simulink model "gm_test_phase_voltages_without_delays"  (R2022a)
settings: Solver=FixedStepDiscrete  StartTime=0.0  StopTime=10.0  RelTol=1e-3
undefined symbols (not defined in the file or in its folder): f_c, u_dc
libraries: hdlmdlgenlib x22, simulink x2
(part 1 of 5)
settings Model: Creator=Andre Merx  LastModifiedBy=Andre Merx
settings SolverCC: AlgebraicLoopSolver=TrustRegion
settings DataIOCC: LimitDataPoints=on  SaveOutput=off  SaveTime=off
settings OptimizationCC: BlockReduction=off  ConditionallyExecuteInputs=off  DefaultParameterBehavior=Inlined  LifeSpan=inf
settings DebuggingCC: AlgebraicLoopMsg=error  InheritedTsInSrcMsg=none  SingleTaskRateTransMsg=error  UnconnectedInputMsg=warning  UnconnectedOutputMsg=warning  UnconnectedLineMsg=warning  AllowSymbolicDim=off  StrictBusMsg=ErrorOnBusTreatedAsVector  SFUnexpectedBacktrackingDiag=warning  SFNoUnconditionalDefaultTransitionDiag=warning  SFExecutionAtInitializationDiag=none  SFMachineParentedDataDiag=warning  ArithmeticOperatorsInVariantConditions=warning
settings HardwareCC: ProdBitPerPointer=32  ProdBitPerSizeT=32  ProdBitPerPtrDiffT=32  ProdLargestAtomicFloat=None  ProdIntDivRoundTo=Undefined  ProdEndianess=Unspecified  ProdWordSize=32  ProdHWDeviceType=ASIC/FPGA->ASIC/FPGA  ProdEqTarget=off
settings SFSimCC: SimUseLocalCustomCode=off  CustomCodeUndefinedFunction=UseInterfaceOnly
settings RTWCC: RTWUseLocalCustomCode=off
settings CodeAppCC: StateflowObjectComments=on
settings GRTTargetCC: TargetLangStandard=C89/C90 (ANSI)
settings ConfigComp: CovScope=ReferencedModels  CovMetricSettings=dw  CovSaveCumulativeToWorkspaceVar=on  CovSaveSingleToWorkspaceVar=on  CovExternalEMLEnable=off  CovSFcnEnable=off

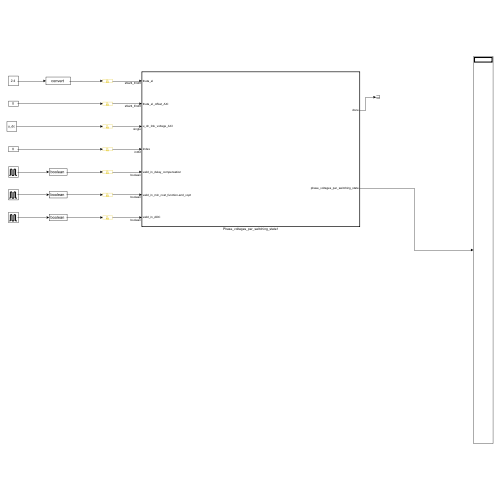
[thumbnail: Simulink's stored preview of the top-level diagram]
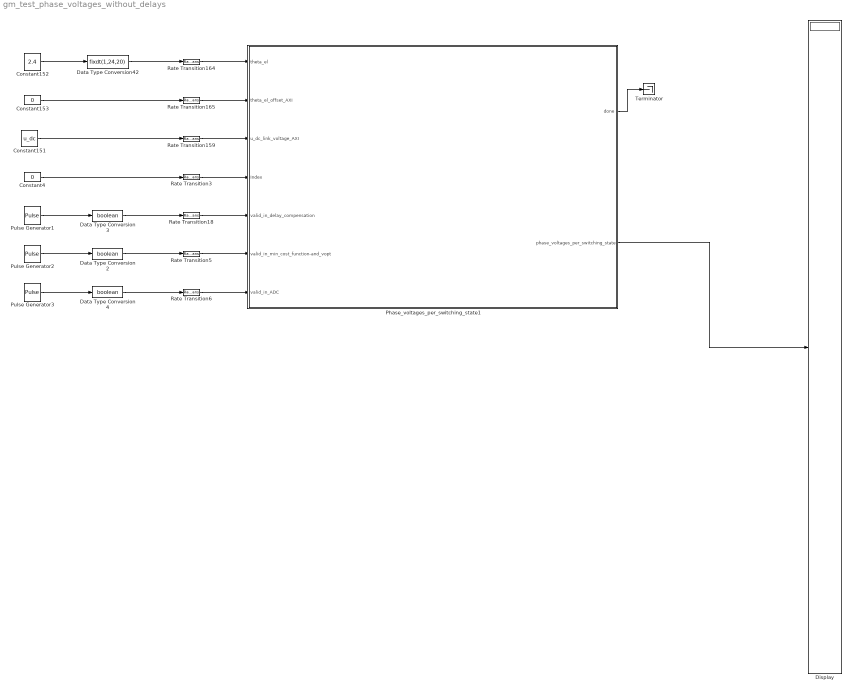
== system gm_test_phase_voltages_without_delays ==
  Constant151 : Constant  Value=u_dc  OutDataTypeStr=single  SampleTime=-1
  Constant152 : Constant  Value=2.4
  Constant153 : Constant  Value=0  OutDataTypeStr=fixdt(1,24,20)  SampleTime=-1
  Constant4 : Constant  Value=0  OutDataTypeStr=int32  SampleTime=-1
  Data Type Conversion2 : DataTypeConversion  OutDataTypeStr=boolean  SaturateOnIntegerOverflow=off  RndMeth=Floor
  Data Type Conversion3 : DataTypeConversion  OutDataTypeStr=boolean  SaturateOnIntegerOverflow=off  RndMeth=Floor
  Data Type Conversion4 : DataTypeConversion  OutDataTypeStr=boolean  SaturateOnIntegerOverflow=off  RndMeth=Floor
  Data Type Conversion42 : DataTypeConversion  OutDataTypeStr=fixdt(1,24,20)  SaturateOnIntegerOverflow=off  RndMeth=Floor
  Display : Display
  Phase_voltages_per_switching_state1 : Subsystem  TreatAsAtomicUnit=on
  Pulse Generator1 : DiscretePulseGenerator  PulseType=Time based  Period=1/f_c
  Pulse Generator2 : DiscretePulseGenerator  PulseType=Time based  Period=1/f_c
  Pulse Generator3 : DiscretePulseGenerator  PulseType=Time based  Period=1/f_c
  Rate Transition{3,5..6,18,159,164..165} (7 alike) : RateTransition  OutPortSampleTime=Rt
  Terminator : Terminator
  wires:
  Phase_voltages_per_switching_state1/2(phase_voltages_per_switching_state) -> Display/1
  Phase_voltages_per_switching_state1/1(done) -> Terminator/1
  Pulse Generator2/1 -> Data Type Conversion2/1
  Rate Transition5/1 -> Phase_voltages_per_switching_state1/6(valid_in_min_cost_function-and_vopt)
  Pulse Generator3/1 -> Data Type Conversion4/1
  Data Type Conversion2/1 -> Rate Transition5/1
  Constant4/1 -> Rate Transition3/1
  Data Type Conversion4/1 -> Rate Transition6/1
  Rate Transition3/1 -> Phase_voltages_per_switching_state1/4(Index)
  Pulse Generator1/1 -> Data Type Conversion3/1
  Rate Transition18/1 -> Phase_voltages_per_switching_state1/5(valid_in_delay_compensation)
  Rate Transition6/1 -> Phase_voltages_per_switching_state1/7(valid_in_ADC)
  Data Type Conversion3/1 -> Rate Transition18/1
  Data Type Conversion42/1 -> Rate Transition164/1
  Constant151/1 -> Rate Transition159/1
  Constant153/1 -> Rate Transition165/1
  Constant152/1 -> Data Type Conversion42/1
  Rate Transition159/1 -> Phase_voltages_per_switching_state1/3(u_dc_link_voltage_AXI)
  Rate Transition164/1 -> Phase_voltages_per_switching_state1/1(theta_el)
  Rate Transition165/1 -> Phase_voltages_per_switching_state1/2(theta_el_offset_AXI)

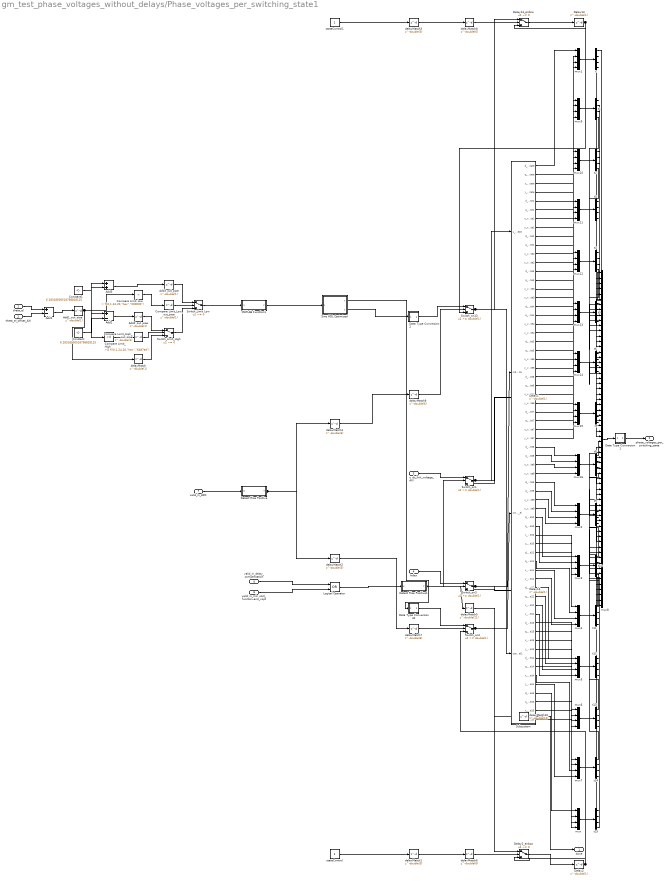
== system gm_test_phase_voltages_without_delays/Phase_voltages_per_switching_state1 ==
  theta_el : Inport  OutDataTypeStr=fixdt(1, 24, 20)  PortDimensions=1  SampleTime=1e-08
  theta_el_offset_AXI : Inport  Port=2  OutDataTypeStr=fixdt(1, 24, 20)  PortDimensions=1  SampleTime=1e-08
  u_dc_link_voltage_AXI : Inport  Port=3  OutDataTypeStr=single  PortDimensions=1  SampleTime=1e-08
  Index : Inport  Port=4  OutDataTypeStr=int32  PortDimensions=1  SampleTime=1e-08
  valid_in_delay_compensation : Inport  Port=5  OutDataTypeStr=boolean  PortDimensions=1  SampleTime=1e-08
  valid_in_min_cost_function-and_vopt : Inport  Port=6  OutDataTypeStr=boolean  PortDimensions=1  SampleTime=1e-08
  valid_in_ADC : Inport  Port=7  OutDataTypeStr=boolean  PortDimensions=1  SampleTime=1e-08
  Add1 : Sum  Inputs=+-  AccumDataTypeStr=fixdt(1, 24, 20)  OutDataTypeStr=fixdt(1, 24, 20)  SampleTime=1e-08
  Add1_out_pipe : Delay  DelayLength=double(1)  InitialCondition=0  SampleTime=1e-08
  Add2 : Sum  Inputs=+-  AccumDataTypeStr=fixdt(1, 24, 20)  OutDataTypeStr=fixdt(1, 24, 20)  SampleTime=1e-08
  Add2_out_pipe : Delay  DelayLength=double(1)  InitialCondition=0  SampleTime=1e-08
  Add3 : Sum  AccumDataTypeStr=fixdt(1, 24, 20)  OutDataTypeStr=fixdt(1, 24, 20)  SampleTime=1e-08
  Add3_out_pipe : Delay  DelayLength=double(1)  InitialCondition=0  SampleTime=1e-08
  Compare Limit_High : simulink/Logic and Bit Operations/Compare To Constant  relop=>=  const="fi(0,1,24,20,\"hex\",\"6487ed\")"  OutDataTypeStr=boolean
  Compare Limit_High_out_pipe : Delay  DelayLength=double(1)  InitialCondition=0  SampleTime=1e-08
  Compare Limit_Low : simulink/Logic and Bit Operations/Compare To Constant  relop=<  const="fi(0,1,24,20,\"hex\",\"000000\")"  OutDataTypeStr=boolean
  Compare Limit_Low_out_pipe : Delay  DelayLength=double(1)  InitialCondition=0  SampleTime=1e-08
  Constant : Constant  Value=6.28318500518798828125  OutDataTypeStr=fixdt(1, 24, 20)  SampleTime=1e-08
  Constant1 : Constant  Value=6.28318500518798828125  OutDataTypeStr=fixdt(1, 24, 20)  SampleTime=1e-08
  Data Type Conversion1 : Subsystem
      mask Display: disp('NFP\nconv');
  Data Type Conversion2 : Subsystem
      mask Display: disp('NFP\nconv');
  Data Type Conversion42 : Subsystem
      mask Display: disp('NFP\nconv');
  Delay{1..2,13..14} (4 alike) : Delay  DelayLength=double(1)  InitialCondition=0  SampleTime=1e-08
  Delay13_enbsw : Switch  Criteria=u2 ~= 0  Threshold=double(0)  OutDataTypeStr=single  SampleTime=1e-08  SaturateOnIntegerOverflow=off  InputSameDT=off
  Delay2_enbsw : Switch  Criteria=u2 ~= 0  Threshold=double(0)  OutDataTypeStr=single  SampleTime=1e-08  SaturateOnIntegerOverflow=off  InputSameDT=off
  Detect Rise Positive : Subsystem  mask(Detect Rise Positive){vinit=double(0), InputProcessing=Elements as channels (sample based), OutDataTypeStr=boolean}
      mask prompts: vinit "Simulink:masks:InitialCondition_MP"; InputProcessing "Simulink:masks:InputProcessing_MP"; OutDataTypeStr "Simulink:masks:OutputDataType_MP"
      mask help: Simulink:masks:DetectRisePositive_MD
      mask init:
      | InputProcessing = 'Elements as channels (sample based)';
      | OutDataTypeStr = 'boolean';
      | vinit = double(0);
      mask TypeOptions InputProcessing: Simulink:masks:ColumnsAsChannelsFrameBased | Simulink:masks:ElementsAsChannelsSampleBased
      mask TypeOptions OutDataTypeStr: Simulink:masks:uint8 | Simulink:masks:boolean
      mask Display: fprintf('U > 0\n&  NOT\nU/z > 0')
  Detect Rise Positive1 : Subsystem  mask(Detect Rise Positive){vinit=double(0), InputProcessing=Elements as channels (sample based), OutDataTypeStr=boolean}
      mask prompts: vinit "Simulink:masks:InitialCondition_MP"; InputProcessing "Simulink:masks:InputProcessing_MP"; OutDataTypeStr "Simulink:masks:OutputDataType_MP"
      mask help: Simulink:masks:DetectRisePositive_MD
      mask init:
      | InputProcessing = 'Elements as channels (sample based)';
      | OutDataTypeStr = 'boolean';
      | vinit = double(0);
      mask TypeOptions InputProcessing: Simulink:masks:ColumnsAsChannelsFrameBased | Simulink:masks:ElementsAsChannelsSampleBased
      mask TypeOptions OutDataTypeStr: Simulink:masks:uint8 | Simulink:masks:boolean
      mask Display: fprintf('U > 0\n&  NOT\nU/z > 0')
  Logical Operator : Logic  Operator=OR  AllPortsSameDT=off  OutDataTypeStr=boolean  SampleTime=1e-08
  MATLAB Function1 : Subsystem
  Sine HDL Optimized : Subsystem  mask(Sine and Cosine HDL optimized block){OutputFormula=sin(2*pi*u) and cos(2*pi*u), NumDataPoints=double(64), TableDataTypeStr=fixdt(1,24,20), SimulateLUTROMDelay=off}
      mask prompts: OutputFormula "Simulink:masks:OutputFormula_MP"; NumDataPoints "HDLShared:hdlshared:CosineHDL_Npts"; TableDataTypeStr "Simulink:blkprm_prompts:TABLE_UNIFIEDDATATYPE"; SimulateLUTROMDelay "HDLShared:hdlshared:CosineHDL_SimulateLUTDelay"
      mask help: Sine and Cosine HDL optimized block using quarter wave symmetry, and HDL friendly settings.
      mask Help: helpview([docroot '/hdlcoder/helptargets.map'],'SineAndCosineHDL_Optimized');
      mask TypeOptions OutputFormula: sin(2*pi*u) | cos(2*pi*u) | exp(j*2*pi*u) | sin(2*pi*u) and cos(2*pi*u)
      mask Display:
      | port_label('input',1,'u')
      | port_label('output',1,'sin(2*pi*u)')
      | port_label('output',2,'cos(2*pi*u)')
      | xpos = 0.35;
      | yoffset = 0.5;
      | if ( SimulateLUTROMDelay )
      |   text(xpos,yoffset,'HDL (Z^{-1})','texmode','on')
      | else
      |    text(xpos,yoffset,'HDL')
      | end
  Subsystem : Subsystem
  Switch_Limit_High : Switch  Criteria=u2 ~= 0  Threshold=double(0)  OutDataTypeStr=fixdt(1, 24, 20)  SampleTime=1e-08  SaturateOnIntegerOverflow=off  InputSameDT=off
  Switch_Limit_Low : Switch  Criteria=u2 ~= 0  Threshold=double(0)  OutDataTypeStr=fixdt(1, 24, 20)  SampleTime=1e-08  SaturateOnIntegerOverflow=off  InputSameDT=off
  Switch_on1 : Switch  Threshold=double(1)  OutDataTypeStr=single  RndMeth=Simplest  SampleTime=1e-08  SaturateOnIntegerOverflow=off  InputSameDT=off
  Switch_on13 : Switch  Threshold=double(1)  OutDataTypeStr=single  RndMeth=Simplest  SampleTime=1e-08  SaturateOnIntegerOverflow=off  InputSameDT=off
  Switch_on2 : Switch  Threshold=double(1)  OutDataTypeStr=single  RndMeth=Simplest  SampleTime=1e-08  SaturateOnIntegerOverflow=off  InputSameDT=off
  Switch_on3 : Switch  Threshold=double(1)  OutDataTypeStr=int32  RndMeth=Simplest  SampleTime=1e-08  SaturateOnIntegerOverflow=off  InputSameDT=off
  delayMatch : Delay  DelayLength=double(1)  InitialCondition=0  SampleTime=1e-08
  delayMatch{1..4} (4 alike) : Delay  DelayLength=double(3)  InitialCondition=0  SampleTime=1e-08
  delayMatch10 : Delay  DelayLength=double(12)  InitialCondition=0  SampleTime=1e-08
  delayMatch5 : Delay  DelayLength=double(21)  InitialCondition=0  SampleTime=1e-08
  delayMatch{6..9} (4 alike) : Delay  DelayLength=double(6)  InitialCondition=0  SampleTime=1e-08
  mux{,1..7,9..16} (16 alike) : Mux
  mux8 : Mux  Inputs=64
  stateControl : Constant  OutDataTypeStr=boolean  SampleTime=1e-08
  stateControl1 : Constant  OutDataTypeStr=boolean  SampleTime=1e-08
  t{,1..15} (16 alike) : Demux
  done : Outport  SampleTime=1e-08
  phase_voltages_per_switching_state : Outport  Port=2  SampleTime=1e-08
  wires:
  theta_el/1 -> Add1/1
  theta_el_offset_AXI/1 -> Add1/2
  u_dc_link_voltage_AXI/1 -> Switch_on1/1
  Index/1 -> Switch_on3/1
  valid_in_delay_compensation/1 -> Logical Operator/1
  valid_in_min_cost_function-and_vopt/1 -> Logical Operator/2
  valid_in_ADC/1 -> Detect Rise Positive/1(U)
  delayMatch/1 -> Switch_Limit_High/3
  Add2_out_pipe/1 -> Switch_Limit_High/1
  Add3_out_pipe/1 -> Switch_Limit_Low/1
  Compare Limit_High_out_pipe/1 -> Switch_Limit_High/2
  Compare Limit_Low_out_pipe/1 -> Switch_Limit_Low/2
  Constant/1 -> Add2/2
  Constant1/1 -> Add3/2
  delayMatch7/1 -> Switch_on2/2
  delayMatch10/1 -> done/1
  Logical Operator/1 -> Detect Rise Positive1/1(U)
  MATLAB Function1/1(y) -> Sine HDL Optimized/1(u)
  mux/1 -> t15/1
  mux1/1 -> t/1
  mux2/1 -> t9/1
  mux3/1 -> t10/1
  mux4/1 -> t11/1
  mux5/1 -> t12/1
  mux6/1 -> t13/1
  mux7/1 -> t14/1
  mux8/1 -> Data Type Conversion1/1(In1)
  mux9/1 -> t1/1
  mux10/1 -> t2/1
  mux11/1 -> t3/1
  mux12/1 -> t4/1
  mux13/1 -> t5/1
  mux14/1 -> t6/1
  mux15/1 -> t7/1
  mux16/1 -> t8/1
  Sine HDL Optimized/1(x) -> Data Type Conversion42/1(In1)
  Sine HDL Optimized/2(y) -> Data Type Conversion2/1(In1)
  Subsystem/1(d_voltage_per_switching_state) -> mux1/1
  Subsystem/2(q_voltage_per_switching_state) -> mux1/2
  Subsystem/3(x_voltage_per_switching_state) -> mux1/3
  Subsystem/4(y_voltage_per_switching_state) -> mux1/4
  Subsystem/5(d_voltage_per_switching_state1) -> mux9/1
  Subsystem/6(q_voltage_per_switching_state1) -> mux9/2
  Subsystem/7(x_voltage_per_switching_state1) -> mux9/3
  Subsystem/8(y_voltage_per_switching_state1) -> mux9/4
  Subsystem/9(d_voltage_per_switching_state2) -> mux10/1
  Subsystem/10(q_voltage_per_switching_state2) -> mux10/2
  Subsystem/11(x_voltage_per_switching_state2) -> mux10/3
  Subsystem/12(y_voltage_per_switching_state2) -> mux10/4
  Subsystem/13(d_voltage_per_switching_state3) -> mux11/1
  Subsystem/14(q_voltage_per_switching_state3) -> mux11/2
  Subsystem/15(x_voltage_per_switching_state3) -> mux11/3
  Subsystem/16(y_voltage_per_switching_state3) -> mux11/4
  Subsystem/17(d_voltage_per_switching_state4) -> mux12/1
  Subsystem/18(q_voltage_per_switching_state4) -> mux12/2
  Subsystem/19(x_voltage_per_switching_state4) -> mux12/3
  Subsystem/20(y_voltage_per_switching_state4) -> mux12/4
  Subsystem/21(d_voltage_per_switching_state5) -> mux13/1
  Subsystem/22(q_voltage_per_switching_state5) -> mux13/2
  Subsystem/23(x_voltage_per_switching_state5) -> mux13/3
  Subsystem/24(y_voltage_per_switching_state5) -> mux13/4
  Subsystem/25(d_voltage_per_switching_state6) -> mux14/1
  Subsystem/26(q_voltage_per_switching_state6) -> mux14/2
  Subsystem/27(x_voltage_per_switching_state6) -> mux14/3
  Subsystem/28(y_voltage_per_switching_state6) -> mux14/4
  Subsystem/29(d_voltage_per_switching_state7) -> mux15/1
  Subsystem/30(q_voltage_per_switching_state7) -> mux15/2
  Subsystem/31(x_voltage_per_switching_state7) -> mux15/3
  Subsystem/32(y_voltage_per_switching_state7) -> mux15/4
  Subsystem/33(d_voltage_per_switching_state8) -> mux16/1
  Subsystem/34(q_voltage_per_switching_state8) -> mux16/2
  Subsystem/35(x_voltage_per_switching_state8) -> mux16/3
  Subsystem/36(y_voltage_per_switching_state8) -> mux16/4
  Subsystem/37(d_voltage_per_switching_state9) -> mux2/1
  Subsystem/38(q_voltage_per_switching_state9) -> mux2/2
  Subsystem/39(x_voltage_per_switching_state9) -> mux2/3
  Subsystem/40(y_voltage_per_switching_state9) -> mux2/4
  Subsystem/41(d_voltage_per_switching_state10) -> mux3/1
  Subsystem/42(q_voltage_per_switching_state10) -> mux3/2
  Subsystem/43(x_voltage_per_switching_state10) -> mux3/3
  Subsystem/44(y_voltage_per_switching_state10) -> mux3/4
  Subsystem/45(d_voltage_per_switching_state11) -> mux4/1
  Subsystem/46(q_voltage_per_switching_state11) -> mux4/2
  Subsystem/47(x_voltage_per_switching_state11) -> mux4/3
  Subsystem/48(y_voltage_per_switching_state11) -> mux4/4
  Subsystem/49(d_voltage_per_switching_state12) -> mux5/1
  Subsystem/50(q_voltage_per_switching_state12) -> mux5/2
  Subsystem/51(x_voltage_per_switching_state12) -> mux5/3
  Subsystem/52(y_voltage_per_switching_state12) -> mux5/4
  Subsystem/53(d_voltage_per_switching_state13) -> mux6/1
  Subsystem/54(q_voltage_per_switching_state13) -> mux6/2
  Subsystem/55(x_voltage_per_switching_state13) -> mux6/3
  Subsystem/56(y_voltage_per_switching_state13) -> mux6/4
  Subsystem/57(d_voltage_per_switching_state14) -> mux7/1
  Subsystem/58(q_voltage_per_switching_state14) -> mux7/2
  Subsystem/59(x_voltage_per_switching_state14) -> mux7/3
  Subsystem/60(y_voltage_per_switching_state14) -> mux7/4
  Subsystem/61(d_voltage_per_switching_state15) -> mux/1
  Subsystem/62(q_voltage_per_switching_state15) -> mux/2
  Subsystem/63(x_voltage_per_switching_state15) -> mux/3
  Subsystem/64(y_voltage_per_switching_state15) -> mux/4
  Switch_Limit_High/1 -> Switch_Limit_Low/3
  Switch_Limit_Low/1 -> MATLAB Function1/1(u)
  Switch_on1/1 -> Subsystem/1(u_dc_link_voltage15), Delay1/1
  Switch_on3/1 -> Subsystem/2(Index 15), Delay14/1
  Add1/1 -> Add1_out_pipe/1
  Add2/1 -> Add2_out_pipe/1
  Add3/1 -> Add3_out_pipe/1
  Compare Limit_High/1 -> Compare Limit_High_out_pipe/1
  Compare Limit_Low/1 -> Compare Limit_Low_out_pipe/1
  t/1 -> mux8/1
  t/2 -> mux8/2
  t/3 -> mux8/3
  t/4 -> mux8/4
  t1/1 -> mux8/5
  t1/2 -> mux8/6
  t1/3 -> mux8/7
  t1/4 -> mux8/8
  t2/1 -> mux8/9
  t2/2 -> mux8/10
  t2/3 -> mux8/11
  t2/4 -> mux8/12
  t3/1 -> mux8/13
  t3/2 -> mux8/14
  t3/3 -> mux8/15
  t3/4 -> mux8/16
  t4/1 -> mux8/17
  t4/2 -> mux8/18
  t4/3 -> mux8/19
  t4/4 -> mux8/20
  t5/1 -> mux8/21
  t5/2 -> mux8/22
  t5/3 -> mux8/23
  t5/4 -> mux8/24
  t6/1 -> mux8/25
  t6/2 -> mux8/26
  t6/3 -> mux8/27
  t6/4 -> mux8/28
  t7/1 -> mux8/29
  t7/2 -> mux8/30
  t7/3 -> mux8/31
  t7/4 -> mux8/32
  t8/1 -> mux8/33
  t8/2 -> mux8/34
  t8/3 -> mux8/35
  t8/4 -> mux8/36
  t9/1 -> mux8/37
  t9/2 -> mux8/38
  t9/3 -> mux8/39
  t9/4 -> mux8/40
  t10/1 -> mux8/41
  t10/2 -> mux8/42
  t10/3 -> mux8/43
  t10/4 -> mux8/44
  t11/1 -> mux8/45
  t11/2 -> mux8/46
  t11/3 -> mux8/47
  t11/4 -> mux8/48
  t12/1 -> mux8/49
  t12/2 -> mux8/50
  t12/3 -> mux8/51
  t12/4 -> mux8/52
  t13/1 -> mux8/53
  t13/2 -> mux8/54
  t13/3 -> mux8/55
  t13/4 -> mux8/56
  t14/1 -> mux8/57
  t14/2 -> mux8/58
  t14/3 -> mux8/59
  t14/4 -> mux8/60
  t15/1 -> mux8/61
  t15/2 -> mux8/62
  t15/3 -> mux8/63
  t15/4 -> mux8/64
  delayMatch6/1 -> Delay2_enbsw/2
  delayMatch8/1 -> Delay13_enbsw/2
  Add1_out_pipe/1 -> delayMatch/1, Compare Limit_Low/1, Compare Limit_High/1, Add3/1, Add2/1
  stateControl/1 -> delayMatch1/1
  delayMatch9/1 -> Switch_on13/2
  stateControl1/1 -> delayMatch3/1
  Detect Rise Positive/1(Y) -> delayMatch4/1, delayMatch2/1
  Detect Rise Positive1/1(Y) -> delayMatch5/1, Switch_on1/2, Switch_on3/2
  Data Type Conversion1/1(Out1) -> phase_voltages_per_switching_state/1
  Data Type Conversion2/1(Out1) -> Switch_on13/1
  Data Type Conversion42/1(Out1) -> Switch_on2/1
  delayMatch1/1 -> delayMatch6/1
  delayMatch2/1 -> delayMatch7/1
  delayMatch3/1 -> delayMatch8/1
  delayMatch4/1 -> delayMatch9/1
  delayMatch5/1 -> delayMatch10/1
  Switch_on2/1 -> Subsystem/3(sin_theta_el), Delay2_enbsw/1
  Switch_on13/1 -> Subsystem/4(cos_theta_el1), Delay13_enbsw/1
  Delay1/1 -> Switch_on1/3
  Delay14/1 -> Switch_on3/3
  Delay2_enbsw/1 -> Delay2/1
  Delay2/1 -> Switch_on2/3, Delay2_enbsw/3
  Delay13_enbsw/1 -> Delay13/1
  Delay13/1 -> Switch_on13/3, Delay13_enbsw/3

== system gm_test_phase_voltages_without_delays/Phase_voltages_per_switching_state1/Data Type Conversion1 ==
  In1 : Inport
  Data Type Conversion1 : DataTypeConversion  OutDataTypeStr=fixdt(1, 24, 11)  SampleTime=1e-08  SaturateOnIntegerOverflow=off  RndMeth=Floor
  Data Type Conversion1_pd1 : Delay  DelayLength=6
  Out1 : Outport
  wires:
  In1/1 -> Data Type Conversion1/1
  Data Type Conversion1/1 -> Data Type Conversion1_pd1/1
  Data Type Conversion1_pd1/1 -> Out1/1

== system gm_test_phase_voltages_without_delays/Phase_voltages_per_switching_state1/Data Type Conversion2 ==
  In1 : Inport
  Data Type Conversion2 : DataTypeConversion  OutDataTypeStr=single  SampleTime=1e-08  SaturateOnIntegerOverflow=off  RndMeth=Floor
  Data Type Conversion2_pd1 : Delay  DelayLength=6
  Out1 : Outport
  wires:
  In1/1 -> Data Type Conversion2/1
  Data Type Conversion2/1 -> Data Type Conversion2_pd1/1
  Data Type Conversion2_pd1/1 -> Out1/1

== system gm_test_phase_voltages_without_delays/Phase_voltages_per_switching_state1/Data Type Conversion42 ==
  In1 : Inport
  Data Type Conversion42 : DataTypeConversion  OutDataTypeStr=single  SampleTime=1e-08  SaturateOnIntegerOverflow=off  RndMeth=Floor
  Data Type Conversion42_pd1 : Delay  DelayLength=6
  Out1 : Outport
  wires:
  In1/1 -> Data Type Conversion42/1
  Data Type Conversion42/1 -> Data Type Conversion42_pd1/1
  Data Type Conversion42_pd1/1 -> Out1/1

== system gm_test_phase_voltages_without_delays/Phase_voltages_per_switching_state1/Detect Rise Positive ==
  note: Edge
  note: U(k)
  U : Inport  OutDataTypeStr=boolean  SampleTime=1e-08
  Delay Input1 : UnitDelay  Description=Store in Global RAM  DisableCoverage=on  InitialCondition=vinit  SampleTime=-1  HasFrameUpgradeWarning=on
  FixPt Relational Operator : RelationalOperator  Operator=>  OutDataTypeStr=boolean  ZeroCross=off  InputSameDT=off
  Positive : Subsystem  mask(Compare To Zero){relop=>, OutDataTypeStr=boolean, ZeroCross=off}
      mask prompts: relop "Simulink:masks:Operator_MP"; OutDataTypeStr "Simulink:masks:OutputDataType_MP"; ZeroCross "Simulink:masks:EnableZerocrossingDetection_MP"
      mask help: Simulink:masks:CompareToZero_MD
      mask init:
      | OutDataTypeStr = 'boolean';
      | ZeroCross = 'off';
      | blkName = 'test_phase_voltages_without_delays/Phase_voltages_per_switching_state1/Detect Rise\nPositive/Positive';
      | relop = '>';
      | setValue = 'boolean';
      mask TypeOptions relop: == | ~= | < | <= | >= | >
      mask TypeOptions OutDataTypeStr: Simulink:masks:uint8 | Simulink:masks:boolean
      mask Callback ZeroCross: sl('zeroCrossEnable', gcbh);
      mask Display: disp([relop,' 0'])
  Y : Outport  SampleTime=1e-08
  wires:
  Delay Input1/1 -> FixPt Relational Operator/2
  FixPt Relational Operator/1 -> Y/1
  Positive/1(y) -> FixPt Relational Operator/1, Delay Input1/1
  U/1 -> Positive/1(u)

== system gm_test_phase_voltages_without_delays/Phase_voltages_per_switching_state1/Detect Rise Positive1 ==
  note: Edge
  note: U(k)
  U : Inport  OutDataTypeStr=boolean  SampleTime=1e-08
  Delay Input1 : UnitDelay  Description=Store in Global RAM  DisableCoverage=on  InitialCondition=vinit  SampleTime=-1  HasFrameUpgradeWarning=on
  FixPt Relational Operator : RelationalOperator  Operator=>  OutDataTypeStr=boolean  ZeroCross=off  InputSameDT=off
  Positive : Subsystem  mask(Compare To Zero){relop=>, OutDataTypeStr=boolean, ZeroCross=off}
      mask prompts: relop "Simulink:masks:Operator_MP"; OutDataTypeStr "Simulink:masks:OutputDataType_MP"; ZeroCross "Simulink:masks:EnableZerocrossingDetection_MP"
      mask help: Simulink:masks:CompareToZero_MD
      mask init:
      | OutDataTypeStr = 'boolean';
      | ZeroCross = 'off';
      | blkName = 'test_phase_voltages_without_delays/Phase_voltages_per_switching_state1/Detect Rise\nPositive1/Positive';
      | relop = '>';
      | setValue = 'boolean';
      mask TypeOptions relop: == | ~= | < | <= | >= | >
      mask TypeOptions OutDataTypeStr: Simulink:masks:uint8 | Simulink:masks:boolean
      mask Callback ZeroCross: sl('zeroCrossEnable', gcbh);
      mask Display: disp([relop,' 0'])
  Y : Outport  SampleTime=1e-08
  wires:
  Delay Input1/1 -> FixPt Relational Operator/2
  FixPt Relational Operator/1 -> Y/1
  Positive/1(y) -> FixPt Relational Operator/1, Delay Input1/1
  U/1 -> Positive/1(u)

== system gm_test_phase_voltages_without_delays/Phase_voltages_per_switching_state1/MATLAB Function1 ==
  u : Inport  OutDataTypeStr=fixdt(1, 24, 20)  PortDimensions=1  SampleTime=1e-08
  MATLAB Function1 : MATLAB Function  TreatAsAtomicUnit=on
  y : Outport  SampleTime=1e-08  VectorParamsAs1DForOutWhenUnconnected=off
  wires:
  MATLAB Function1/1(y) -> y/1
  u/1 -> MATLAB Function1/1(u)

== system gm_test_phase_voltages_without_delays/Phase_voltages_per_switching_state1/Sine HDL Optimized ==
  note: (C) 2016 Mathworks, Inc
  note: (C) 2016 Mathworks, Inc
  u : Inport  OutDataTypeStr=fixdt(1,48,45,'DataTypeOverride', 'Off')  SampleTime=1e-08
  1st or 4th Quad : Logic  Operator=OR  AllPortsSameDT=off  OutDataTypeStr=boolean  SampleTime=1e-08
  Amp25 : Sum  Inputs=+-  AccumDataTypeStr=fixdt(1, 26, 25)  OutDataTypeStr=fixdt(1, 26, 25)  SampleTime=1e-08
  Amp50 : Sum  Inputs=+-  AccumDataTypeStr=fixdt(1, 26, 25)  OutDataTypeStr=fixdt(1, 26, 25)  SampleTime=1e-08
  Amp75 : Sum  Inputs=+-  AccumDataTypeStr=fixdt(1, 26, 25)  OutDataTypeStr=fixdt(1, 26, 25)  SampleTime=1e-08
  CastU16En1 : DataTypeConversion  OutDataTypeStr=uint8  ConvertRealWorld=Stored Integer (SI)  SampleTime=1e-08  SaturateOnIntegerOverflow=off  RndMeth=Floor
  CastU16En2 : DataTypeConversion  OutDataTypeStr=uint8  ConvertRealWorld=Stored Integer (SI)  SampleTime=1e-08  RndMeth=Floor
  CastU16En21 : DataTypeConversion  OutDataTypeStr=uint8  ConvertRealWorld=Stored Integer (SI)  SampleTime=1e-08  SaturateOnIntegerOverflow=off  RndMeth=Floor
  CastU16En3 : DataTypeConversion  OutDataTypeStr=fixdt(0, 9, 0)  SampleTime=1e-08  SaturateOnIntegerOverflow=off  RndMeth=Floor
  CastU16En31 : DataTypeConversion  OutDataTypeStr=uint8  ConvertRealWorld=Stored Integer (SI)  SampleTime=1e-08  RndMeth=Floor
  CastU16En4 : DataTypeConversion  OutDataTypeStr=fixdt(0, 9, 0)  SampleTime=1e-08  SaturateOnIntegerOverflow=off  RndMeth=Floor
  Cosine : hdlmdlgenlib/Buffer
      settings: SourceProductBaseCode=SL
  Cosine1 : hdlmdlgenlib/Buffer
      settings: SourceProductBaseCode=SL
  GTEp75 : RelationalOperator  OutDataTypeStr=boolean  SampleTime=1e-08  InputSameDT=off
  LTEp{25,50,251,501} (4 alike) : RelationalOperator  Operator=<=  OutDataTypeStr=boolean  SampleTime=1e-08  InputSameDT=off
  Look-Up Table : Lookup_n-D  NumberOfTableDimensions=1  BreakpointsForDimension1="fi(\"numerictype\",numerictype(0,8,0),\"fimath\",fimath(\"RoundingMethod\", \"Floor\",\"OverflowAction\", \"Wrap\",\"ProductMode\",\"FullPrecision\",\"SumMode\",\"FullPrecision\"),\"Value\",\"[0 1 2 3 4 5 6 7 8 9 10 11 12 13 14 15 16 17 18 19 20 21 22 23 24 25 26 27 28 29 30 31 32 33 34 35 36 37 38 39 40 41 42 43 44 45 46 47 48 49 50 51 52 53 54 55 56 57 58 59 60 61 62 63]\")"  Table="reshape(fi(\"numerictype\",numerictype(1,25,20),\"fimath\",fimath(\"RoundingMethod\", \"Floor\",\"OverflowAction\", \"Wrap\",\"ProductMode\",\"FullPrecision\",\"SumMode\",\"FullPrecision\"),\"Value\",\"[0;0.02454090118408203125;0.04906749725341796875;0.0735645294189453125;0.0980167388916015625;0.12241077423095703125;0.1467304229736328125;0.17096233367919921875;0.19509029388427734375;0.2191009521484375;0.24298000335693359375;0.26671314239501953125;0.2902851104736328125;0.31368160247802734375;0.33689022064208984375;0.35989475250244140625;0.38268375396728515625;0.4052410125732421875;0.427555084228515625;0.449611663818359375;0.47139644622802734375;0.49289798736572265625;0.514102935791015625;0.5349979400634765625;0.5555706024169921875;0.57580852508544921875;0.595699310302734375;0.61523151397705078125;0.6343936920166015625;0.65317249298095703125;0.67155933380126953125;0.689540863037109375;0.70710659027099609375;0.724246978759765625;0.7409515380859375;0.75720882415771484375;0.77301025390625;0.78834629058837890625;0.8032073974609375;0.817584991455078125;0.83146953582763671875;0.84485340118408203125;0.8577289581298828125;0.870086669921875;0.88192081451416015625;0.8932247161865234375;0.90398883819580078125;0.9142093658447265625;0.9238796234130859375;0.9329929351806640625;0.94154453277587890625;0.949527740478515625;0.95694065093994140625;0.963775634765625;0.97003078460693359375;0.9757022857666015625;0.980785369873046875;0.9852771759033203125;0.98917675018310546875;0.9924793243408203125;0.99518489837646484375;0.99729061126708984375;0.99879550933837890625;0.999698638916015625]\"), [1  64])"  InterpMethod=Flat  ExtrapMethod=Clip  DiagnosticForOutOfRangeInput=Error  SampleTime=1e-08  OutDataTypeStr=fixdt(1, 25, 20)
  Look-Up Table1 : Lookup_n-D  NumberOfTableDimensions=1  BreakpointsForDimension1="fi(\"numerictype\",numerictype(0,8,0),\"fimath\",fimath(\"RoundingMethod\", \"Floor\",\"OverflowAction\", \"Wrap\",\"ProductMode\",\"FullPrecision\",\"SumMode\",\"FullPrecision\"),\"Value\",\"[0 1 2 3 4 5 6 7 8 9 10 11 12 13 14 15 16 17 18 19 20 21 22 23 24 25 26 27 28 29 30 31 32 33 34 35 36 37 38 39 40 41 42 43 44 45 46 47 48 49 50 51 52 53 54 55 56 57 58 59 60 61 62 63]\")"  Table="reshape(fi(\"numerictype\",numerictype(1,25,20),\"fimath\",fimath(\"RoundingMethod\", \"Floor\",\"OverflowAction\", \"Wrap\",\"ProductMode\",\"FullPrecision\",\"SumMode\",\"FullPrecision\"),\"Value\",\"[0;0.02454090118408203125;0.04906749725341796875;0.0735645294189453125;0.0980167388916015625;0.12241077423095703125;0.1467304229736328125;0.17096233367919921875;0.19509029388427734375;0.2191009521484375;0.24298000335693359375;0.26671314239501953125;0.2902851104736328125;0.31368160247802734375;0.33689022064208984375;0.35989475250244140625;0.38268375396728515625;0.4052410125732421875;0.427555084228515625;0.449611663818359375;0.47139644622802734375;0.49289798736572265625;0.514102935791015625;0.5349979400634765625;0.5555706024169921875;0.57580852508544921875;0.595699310302734375;0.61523151397705078125;0.6343936920166015625;0.65317249298095703125;0.67155933380126953125;0.689540863037109375;0.70710659027099609375;0.724246978759765625;0.7409515380859375;0.75720882415771484375;0.77301025390625;0.78834629058837890625;0.8032073974609375;0.817584991455078125;0.83146953582763671875;0.84485340118408203125;0.8577289581298828125;0.870086669921875;0.88192081451416015625;0.8932247161865234375;0.90398883819580078125;0.9142093658447265625;0.9238796234130859375;0.9329929351806640625;0.94154453277587890625;0.949527740478515625;0.95694065093994140625;0.963775634765625;0.97003078460693359375;0.9757022857666015625;0.980785369873046875;0.9852771759033203125;0.98917675018310546875;0.9924793243408203125;0.99518489837646484375;0.99729061126708984375;0.99879550933837890625;0.999698638916015625]\"), [1  64])"  InterpMethod=Flat  ExtrapMethod=Clip  DiagnosticForOutOfRangeInput=Error  SampleTime=1e-08  OutDataTypeStr=fixdt(1, 25, 20)
  Negate : UnaryMinus  SampleTime=1e-08
  Negate1 : UnaryMinus  SampleTime=1e-08
  PipelineRegister : Delay  DelayLength=double(1)  InitialCondition=0  SampleTime=1e-08
  PipelineRegister1 : Delay  DelayLength=double(1)  InitialCondition=0  SampleTime=1e-08
  Point25 : Constant  Value=0.25  OutDataTypeStr=fixdt(0, 25, 25)  SampleTime=1e-08
  Point251 : Constant  Value=0.25  OutDataTypeStr=fixdt(0, 25, 25)  SampleTime=1e-08
  Point50 : Constant  Value=0.5  OutDataTypeStr=fixdt(0, 25, 25)  SampleTime=1e-08
  Point501 : Constant  Value=0.5  OutDataTypeStr=fixdt(0, 25, 25)  SampleTime=1e-08
  Point75 : Constant  Value=0.75  OutDataTypeStr=fixdt(0, 25, 25)  SampleTime=1e-08
  Positive : DataTypeConversion  OutDataTypeStr=fixdt(1, 25, 20)  SampleTime=1e-08  SaturateOnIntegerOverflow=off  RndMeth=Floor
  Positive1 : DataTypeConversion  OutDataTypeStr=fixdt(1, 25, 20)  SampleTime=1e-08  SaturateOnIntegerOverflow=off  RndMeth=Floor
  QuadHandle1 : Switch  Criteria=u2 ~= 0  Threshold=double(0)  OutDataTypeStr=fixdt(1, 26, 25)  SampleTime=1e-08  SaturateOnIntegerOverflow=off  InputSameDT=off
  QuadHandle1a : Switch  Criteria=u2 ~= 0  Threshold=double(0)  OutDataTypeStr=fixdt(1, 26, 25)  SampleTime=1e-08  SaturateOnIntegerOverflow=off  InputSameDT=off
  QuadHandle1b : Switch  Criteria=u2 ~= 0  Threshold=double(0)  OutDataTypeStr=fixdt(1, 26, 25)  SampleTime=1e-08  SaturateOnIntegerOverflow=off  InputSameDT=off
  QuadHandle2 : Switch  Criteria=u2 ~= 0  Threshold=double(0)  OutDataTypeStr=fixdt(0, 8, 8)  SampleTime=1e-08  InputSameDT=off
  QuadHandle21 : Switch  Criteria=u2 ~= 0  Threshold=double(0)  OutDataTypeStr=fixdt(0, 8, 8)  SampleTime=1e-08  SaturateOnIntegerOverflow=off  InputSameDT=off
  RAMDelayBalance : hdlmdlgenlib/Buffer
      settings: SourceProductBaseCode=SL
  RAMDelayBalance1 : hdlmdlgenlib/Buffer
      settings: SourceProductBaseCode=SL
  Saturation : Saturate  UpperLimit="fi(0,0,8,0,\"hex\",\"3f\")"  LowerLimit="fi(0,0,8,0,\"hex\",\"00\")"  SampleTime=1e-08  OutDataTypeStr=uint8
  Saturation1 : Saturate  UpperLimit="fi(0,0,8,0,\"hex\",\"3f\")"  LowerLimit="fi(0,0,8,0,\"hex\",\"00\")"  SampleTime=1e-08  OutDataTypeStr=uint8
  SignCorrected : Switch  Criteria=u2 ~= 0  Threshold=double(0)  OutDataTypeStr=fixdt(1, 25, 20)  SampleTime=1e-08  SaturateOnIntegerOverflow=off  InputSameDT=off
  SignCorrected1 : Switch  Criteria=u2 ~= 0  Threshold=double(0)  OutDataTypeStr=fixdt(1, 25, 20)  SampleTime=1e-08  SaturateOnIntegerOverflow=off  InputSameDT=off
  Sine : hdlmdlgenlib/Buffer
      settings: SourceProductBaseCode=SL
  Sine1 : hdlmdlgenlib/Buffer
      settings: SourceProductBaseCode=SL
  Switch : Switch  Criteria=u2 ~= 0  Threshold=double(0)  OutDataTypeStr=uint8  SampleTime=1e-08  SaturateOnIntegerOverflow=off  InputSameDT=off
  Switch1 : Switch  Criteria=u2 ~= 0  Threshold=double(0)  OutDataTypeStr=uint8  SampleTime=1e-08  SaturateOnIntegerOverflow=off  InputSameDT=off
  delayMatch : Delay  DelayLength=double(1)  InitialCondition=0  SampleTime=1e-08
  delayMatch1 : Delay  DelayLength=double(1)  InitialCondition=0  SampleTime=1e-08
  dtc : DataTypeConversion  OutDataTypeStr=uint8  SampleTime=1e-08  SaturateOnIntegerOverflow=off  RndMeth=Floor
  insig : DataTypeConversion  OutDataTypeStr=fixdt(0, 8, 8)  SampleTime=1e-08  SaturateOnIntegerOverflow=off  RndMeth=Floor
  insig1 : DataTypeConversion  OutDataTypeStr=fixdt(0, 8, 8)  SampleTime=1e-08  SaturateOnIntegerOverflow=off  RndMeth=Floor
  p25mA : Sum  Inputs=+-  AccumDataTypeStr=fixdt(1, 26, 25)  OutDataTypeStr=fixdt(1, 26, 25)  SampleTime=1e-08
  p50mA : Sum  Inputs=+-  AccumDataTypeStr=fixdt(1, 27, 25)  OutDataTypeStr=fixdt(1, 27, 25)  SampleTime=1e-08
  p75mA : Sum  Inputs=+-  AccumDataTypeStr=fixdt(1, 26, 25)  OutDataTypeStr=fixdt(1, 26, 25)  SampleTime=1e-08
  pow2switch : Constant  OutDataTypeStr=boolean  SampleTime=1e-08
  pow2switch1 : Constant  OutDataTypeStr=boolean  SampleTime=1e-08
  x : Outport  SampleTime=1e-08
  y : Outport  Port=2  SampleTime=1e-08
  wires:
  Sine1/1 -> x/1
  Cosine1/1 -> y/1
  Cosine/1 -> Cosine1/1
  Sine/1 -> Sine1/1
  dtc/1 -> RAMDelayBalance/1
  Amp25/1 -> QuadHandle1a/3
  Amp75/1 -> QuadHandle1b/1
  CastU16En1/1 -> CastU16En3/1
  CastU16En2/1 -> Switch/3, Saturation/1
  CastU16En3/1 -> CastU16En2/1
  GTEp75/1 -> QuadHandle1b/2, 1st or 4th Quad/2
  LTEp25/1 -> QuadHandle1a/2, 1st or 4th Quad/1
  LTEp50/1 -> QuadHandle2/2
  PipelineRegister/1 -> Positive/1, Negate/1
  Negate/1 -> SignCorrected/3
  Point25/1 -> p25mA/1, LTEp25/2, Amp25/2
  Point50/1 -> LTEp50/2
  Point75/1 -> p75mA/1, GTEp75/2, Amp75/2
  Positive/1 -> SignCorrected/1
  QuadHandle1a/1 -> QuadHandle2/1
  QuadHandle1b/1 -> QuadHandle2/3
  QuadHandle2/1 -> CastU16En1/1
  delayMatch1/1 -> SignCorrected/2
  Saturation/1 -> Switch/1
  SignCorrected/1 -> Cosine/1
  Switch/1 -> Look-Up Table/1
  insig/1 -> p75mA/2, p25mA/2, LTEp50/1, LTEp25/1, GTEp75/1, Amp75/1, Amp25/1
  p25mA/1 -> QuadHandle1a/1
  p75mA/1 -> QuadHandle1b/3
  pow2switch/1 -> Switch/2
  Amp50/1 -> QuadHandle1/3
  CastU16En21/1 -> CastU16En4/1
  CastU16En31/1 -> Switch1/3, Saturation1/1
  CastU16En4/1 -> CastU16En31/1
  LTEp251/1 -> QuadHandle21/2
  LTEp501/1 -> QuadHandle1/2, RAMDelayBalance1/1
  PipelineRegister1/1 -> Positive1/1, Negate1/1
  Negate1/1 -> SignCorrected1/3
  Point251/1 -> LTEp251/2
  Point501/1 -> p50mA/1, LTEp501/2, Amp50/2
  Positive1/1 -> SignCorrected1/1
  QuadHandle1/1 -> p50mA/2, QuadHandle21/1, LTEp251/1
  QuadHandle21/1 -> CastU16En21/1
  delayMatch/1 -> SignCorrected1/2
  Saturation1/1 -> Switch1/1
  SignCorrected1/1 -> Sine/1
  Switch1/1 -> Look-Up Table1/1
  insig1/1 -> QuadHandle1/1, LTEp501/1, Amp50/1
  p50mA/1 -> QuadHandle21/3
  pow2switch1/1 -> Switch1/2
  1st or 4th Quad/1 -> dtc/1
  RAMDelayBalance1/1 -> delayMatch/1
  RAMDelayBalance/1 -> delayMatch1/1
  u/1 -> insig1/1, insig/1
  Look-Up Table/1 -> PipelineRegister/1
  Look-Up Table1/1 -> PipelineRegister1/1

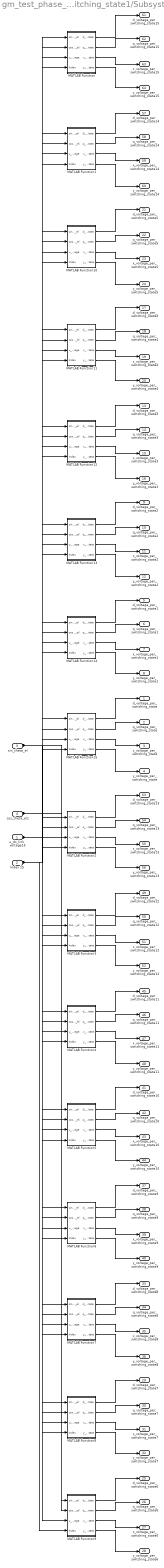
== system gm_test_phase_voltages_without_delays/Phase_voltages_per_switching_state1/Subsystem ==
  u_dc_link_voltage15 : Inport  OutDataTypeStr=single  PortDimensions=1  SampleTime=1e-08
  Index 15 : Inport  Port=2  OutDataTypeStr=int32  PortDimensions=1  SampleTime=1e-08
  sin_theta_el : Inport  Port=3  OutDataTypeStr=single  PortDimensions=1  SampleTime=1e-08
  cos_theta_el1 : Inport  Port=4  OutDataTypeStr=single  PortDimensions=1  SampleTime=1e-08
  MATLAB Function : Subsystem
  MATLAB Function1 : Subsystem
  MATLAB Function10 : Subsystem
  MATLAB Function11 : Subsystem
  MATLAB Function12 : Subsystem
  MATLAB Function13 : Subsystem
  MATLAB Function14 : Subsystem
  MATLAB Function15 : Subsystem
  MATLAB Function2 : Subsystem
  MATLAB Function3 : Subsystem
  MATLAB Function4 : Subsystem
  MATLAB Function5 : Subsystem
  MATLAB Function6 : Subsystem
  MATLAB Function7 : Subsystem
  MATLAB Function8 : Subsystem
  MATLAB Function9 : Subsystem
  d_voltage_per_switching_state : Outport  SampleTime=1e-08
  q_voltage_per_switching_state : Outport  Port=2  SampleTime=1e-08
  x_voltage_per_switching_state : Outport  Port=3  SampleTime=1e-08
  y_voltage_per_switching_state : Outport  Port=4  SampleTime=1e-08
  d_voltage_per_switching_state1 : Outport  Port=5  SampleTime=1e-08
  q_voltage_per_switching_state1 : Outport  Port=6  SampleTime=1e-08
  x_voltage_per_switching_state1 : Outport  Port=7  SampleTime=1e-08
  y_voltage_per_switching_state1 : Outport  Port=8  SampleTime=1e-08
  d_voltage_per_switching_state2 : Outport  Port=9  SampleTime=1e-08
  q_voltage_per_switching_state2 : Outport  Port=10  SampleTime=1e-08
  x_voltage_per_switching_state2 : Outport  Port=11  SampleTime=1e-08
  y_voltage_per_switching_state2 : Outport  Port=12  SampleTime=1e-08
  d_voltage_per_switching_state3 : Outport  Port=13  SampleTime=1e-08
  q_voltage_per_switching_state3 : Outport  Port=14  SampleTime=1e-08
  x_voltage_per_switching_state3 : Outport  Port=15  SampleTime=1e-08
  y_voltage_per_switching_state3 : Outport  Port=16  SampleTime=1e-08
  d_voltage_per_switching_state4 : Outport  Port=17  SampleTime=1e-08
  q_voltage_per_switching_state4 : Outport  Port=18  SampleTime=1e-08
  x_voltage_per_switching_state4 : Outport  Port=19  SampleTime=1e-08
  y_voltage_per_switching_state4 : Outport  Port=20  SampleTime=1e-08
  d_voltage_per_switching_state5 : Outport  Port=21  SampleTime=1e-08
  q_voltage_per_switching_state5 : Outport  Port=22  SampleTime=1e-08
  x_voltage_per_switching_state5 : Outport  Port=23  SampleTime=1e-08
  y_voltage_per_switching_state5 : Outport  Port=24  SampleTime=1e-08
  d_voltage_per_switching_state6 : Outport  Port=25  SampleTime=1e-08
  q_voltage_per_switching_state6 : Outport  Port=26  SampleTime=1e-08
  x_voltage_per_switching_state6 : Outport  Port=27  SampleTime=1e-08
  y_voltage_per_switching_state6 : Outport  Port=28  SampleTime=1e-08
  d_voltage_per_switching_state7 : Outport  Port=29  SampleTime=1e-08
  q_voltage_per_switching_state7 : Outport  Port=30  SampleTime=1e-08
  x_voltage_per_switching_state7 : Outport  Port=31  SampleTime=1e-08
  y_voltage_per_switching_state7 : Outport  Port=32  SampleTime=1e-08
  d_voltage_per_switching_state8 : Outport  Port=33  SampleTime=1e-08
  q_voltage_per_switching_state8 : Outport  Port=34  SampleTime=1e-08
  x_voltage_per_switching_state8 : Outport  Port=35  SampleTime=1e-08
  y_voltage_per_switching_state8 : Outport  Port=36  SampleTime=1e-08
  d_voltage_per_switching_state9 : Outport  Port=37  SampleTime=1e-08
  q_voltage_per_switching_state9 : Outport  Port=38  SampleTime=1e-08
  x_voltage_per_switching_state9 : Outport  Port=39  SampleTime=1e-08
  y_voltage_per_switching_state9 : Outport  Port=40  SampleTime=1e-08
  d_voltage_per_switching_state10 : Outport  Port=41  SampleTime=1e-08
  q_voltage_per_switching_state10 : Outport  Port=42  SampleTime=1e-08
  x_voltage_per_switching_state10 : Outport  Port=43  SampleTime=1e-08
  y_voltage_per_switching_state10 : Outport  Port=44  SampleTime=1e-08
  d_voltage_per_switching_state11 : Outport  Port=45  SampleTime=1e-08
  q_voltage_per_switching_state11 : Outport  Port=46  SampleTime=1e-08
  x_voltage_per_switching_state11 : Outport  Port=47  SampleTime=1e-08
  y_voltage_per_switching_state11 : Outport  Port=48  SampleTime=1e-08
  d_voltage_per_switching_state12 : Outport  Port=49  SampleTime=1e-08
  q_voltage_per_switching_state12 : Outport  Port=50  SampleTime=1e-08
  x_voltage_per_switching_state12 : Outport  Port=51  SampleTime=1e-08
  y_voltage_per_switching_state12 : Outport  Port=52  SampleTime=1e-08
  d_voltage_per_switching_state13 : Outport  Port=53  SampleTime=1e-08
  q_voltage_per_switching_state13 : Outport  Port=54  SampleTime=1e-08
  x_voltage_per_switching_state13 : Outport  Port=55  SampleTime=1e-08
  y_voltage_per_switching_state13 : Outport  Port=56  SampleTime=1e-08
  d_voltage_per_switching_state14 : Outport  Port=57  SampleTime=1e-08
  q_voltage_per_switching_state14 : Outport  Port=58  SampleTime=1e-08
  x_voltage_per_switching_state14 : Outport  Port=59  SampleTime=1e-08
  y_voltage_per_switching_state14 : Outport  Port=60  SampleTime=1e-08
  d_voltage_per_switching_state15 : Outport  Port=61  SampleTime=1e-08
  q_voltage_per_switching_state15 : Outport  Port=62  SampleTime=1e-08
  x_voltage_per_switching_state15 : Outport  Port=63  SampleTime=1e-08
  y_voltage_per_switching_state15 : Outport  Port=64  SampleTime=1e-08
  wires:
  MATLAB Function/1(d_voltage_per_switching_state) -> d_voltage_per_switching_state15/1
  MATLAB Function/2(q_voltage_per_switching_state) -> q_voltage_per_switching_state15/1
  MATLAB Function/3(x_voltage_per_switching_state) -> x_voltage_per_switching_state15/1
  MATLAB Function/4(y_voltage_per_switching_state) -> y_voltage_per_switching_state15/1
  MATLAB Function1/1(d_voltage_per_switching_state) -> d_voltage_per_switching_state14/1
  MATLAB Function1/2(q_voltage_per_switching_state) -> q_voltage_per_switching_state14/1
  MATLAB Function1/3(x_voltage_per_switching_state) -> x_voltage_per_switching_state14/1
  MATLAB Function1/4(y_voltage_per_switching_state) -> y_voltage_per_switching_state14/1
  MATLAB Function10/1(d_voltage_per_switching_state) -> d_voltage_per_switching_state5/1
  MATLAB Function10/2(q_voltage_per_switching_state) -> q_voltage_per_switching_state5/1
  MATLAB Function10/3(x_voltage_per_switching_state) -> x_voltage_per_switching_state5/1
  MATLAB Function10/4(y_voltage_per_switching_state) -> y_voltage_per_switching_state5/1
  MATLAB Function11/1(d_voltage_per_switching_state) -> d_voltage_per_switching_state4/1
  MATLAB Function11/2(q_voltage_per_switching_state) -> q_voltage_per_switching_state4/1
  MATLAB Function11/3(x_voltage_per_switching_state) -> x_voltage_per_switching_state4/1
  MATLAB Function11/4(y_voltage_per_switching_state) -> y_voltage_per_switching_state4/1
  MATLAB Function12/1(d_voltage_per_switching_state) -> d_voltage_per_switching_state3/1
  MATLAB Function12/2(q_voltage_per_switching_state) -> q_voltage_per_switching_state3/1
  MATLAB Function12/3(x_voltage_per_switching_state) -> x_voltage_per_switching_state3/1
  MATLAB Function12/4(y_voltage_per_switching_state) -> y_voltage_per_switching_state3/1
  MATLAB Function13/1(d_voltage_per_switching_state) -> d_voltage_per_switching_state2/1
  MATLAB Function13/2(q_voltage_per_switching_state) -> q_voltage_per_switching_state2/1
  MATLAB Function13/3(x_voltage_per_switching_state) -> x_voltage_per_switching_state2/1
  MATLAB Function13/4(y_voltage_per_switching_state) -> y_voltage_per_switching_state2/1
  MATLAB Function14/1(d_voltage_per_switching_state) -> d_voltage_per_switching_state1/1
  MATLAB Function14/2(q_voltage_per_switching_state) -> q_voltage_per_switching_state1/1
  MATLAB Function14/3(x_voltage_per_switching_state) -> x_voltage_per_switching_state1/1
  MATLAB Function14/4(y_voltage_per_switching_state) -> y_voltage_per_switching_state1/1
  MATLAB Function15/1(d_voltage_per_switching_state) -> d_voltage_per_switching_state/1
  MATLAB Function15/2(q_voltage_per_switching_state) -> q_voltage_per_switching_state/1
  MATLAB Function15/3(x_voltage_per_switching_state) -> x_voltage_per_switching_state/1
  MATLAB Function15/4(y_voltage_per_switching_state) -> y_voltage_per_switching_state/1
  MATLAB Function2/1(d_voltage_per_switching_state) -> d_voltage_per_switching_state13/1
  MATLAB Function2/2(q_voltage_per_switching_state) -> q_voltage_per_switching_state13/1
  MATLAB Function2/3(x_voltage_per_switching_state) -> x_voltage_per_switching_state13/1
  MATLAB Function2/4(y_voltage_per_switching_state) -> y_voltage_per_switching_state13/1
  MATLAB Function3/1(d_voltage_per_switching_state) -> d_voltage_per_switching_state12/1
  MATLAB Function3/2(q_voltage_per_switching_state) -> q_voltage_per_switching_state12/1
  MATLAB Function3/3(x_voltage_per_switching_state) -> x_voltage_per_switching_state12/1
  MATLAB Function3/4(y_voltage_per_switching_state) -> y_voltage_per_switching_state12/1
  MATLAB Function4/1(d_voltage_per_switching_state) -> d_voltage_per_switching_state11/1
  MATLAB Function4/2(q_voltage_per_switching_state) -> q_voltage_per_switching_state11/1
  MATLAB Function4/3(x_voltage_per_switching_state) -> x_voltage_per_switching_state11/1
  MATLAB Function4/4(y_voltage_per_switching_state) -> y_voltage_per_switching_state11/1
  MATLAB Function5/1(d_voltage_per_switching_state) -> d_voltage_per_switching_state10/1
  MATLAB Function5/2(q_voltage_per_switching_state) -> q_voltage_per_switching_state10/1
  MATLAB Function5/3(x_voltage_per_switching_state) -> x_voltage_per_switching_state10/1
  MATLAB Function5/4(y_voltage_per_switching_state) -> y_voltage_per_switching_state10/1
  MATLAB Function6/1(d_voltage_per_switching_state) -> d_voltage_per_switching_state9/1
  MATLAB Function6/2(q_voltage_per_switching_state) -> q_voltage_per_switching_state9/1
  MATLAB Function6/3(x_voltage_per_switching_state) -> x_voltage_per_switching_state9/1
  MATLAB Function6/4(y_voltage_per_switching_state) -> y_voltage_per_switching_state9/1
  MATLAB Function7/1(d_voltage_per_switching_state) -> d_voltage_per_switching_state8/1
  MATLAB Function7/2(q_voltage_per_switching_state) -> q_voltage_per_switching_state8/1
  MATLAB Function7/3(x_voltage_per_switching_state) -> x_voltage_per_switching_state8/1
  MATLAB Function7/4(y_voltage_per_switching_state) -> y_voltage_per_switching_state8/1
  MATLAB Function8/1(d_voltage_per_switching_state) -> d_voltage_per_switching_state7/1
  MATLAB Function8/2(q_voltage_per_switching_state) -> q_voltage_per_switching_state7/1
  MATLAB Function8/3(x_voltage_per_switching_state) -> x_voltage_per_switching_state7/1
  MATLAB Function8/4(y_voltage_per_switching_state) -> y_voltage_per_switching_state7/1
  MATLAB Function9/1(d_voltage_per_switching_state) -> d_voltage_per_switching_state6/1
  MATLAB Function9/2(q_voltage_per_switching_state) -> q_voltage_per_switching_state6/1
  MATLAB Function9/3(x_voltage_per_switching_state) -> x_voltage_per_switching_state6/1
  MATLAB Function9/4(y_voltage_per_switching_state) -> y_voltage_per_switching_state6/1
  u_dc_link_voltage15/1 -> MATLAB Function9/3(u_dc_link_voltage), MATLAB Function8/3(u_dc_link_voltage), MATLAB Function7/3(u_dc_link_voltage), MATLAB Function6/3(u_dc_link_voltage), MATLAB Function5/3(u_dc_link_voltage), MATLAB Function4/3(u_dc_link_voltage), MATLAB Function3/3(u_dc_link_voltage), MATLAB Function2/3(u_dc_link_voltage), MATLAB Function15/3(u_dc_link_voltage), MATLAB Function14/3(u_dc_link_voltage), MATLAB Function13/3(u_dc_link_voltage), MATLAB Function12/3(u_dc_link_voltage), MATLAB Function11/3(u_dc_link_voltage), MATLAB Function10/3(u_dc_link_voltage), MATLAB Function1/3(u_dc_link_voltage), MATLAB Function/3(u_dc_link_voltage)
  Index 15/1 -> MATLAB Function9/4(Index), MATLAB Function8/4(Index), MATLAB Function7/4(Index), MATLAB Function6/4(Index), MATLAB Function5/4(Index), MATLAB Function4/4(Index), MATLAB Function3/4(Index), MATLAB Function2/4(Index), MATLAB Function15/4(Index), MATLAB Function14/4(Index), MATLAB Function13/4(Index), MATLAB Function12/4(Index), MATLAB Function11/4(Index), MATLAB Function10/4(Index), MATLAB Function1/4(Index), MATLAB Function/4(Index)
  sin_theta_el/1 -> MATLAB Function9/1(sin_theta_el), MATLAB Function8/1(sin_theta_el), MATLAB Function7/1(sin_theta_el), MATLAB Function6/1(sin_theta_el), MATLAB Function5/1(sin_theta_el), MATLAB Function4/1(sin_theta_el), MATLAB Function3/1(sin_theta_el), MATLAB Function2/1(sin_theta_el), MATLAB Function15/1(sin_theta_el), MATLAB Function14/1(sin_theta_el), MATLAB Function13/1(sin_theta_el), MATLAB Function12/1(sin_theta_el), MATLAB Function11/1(sin_theta_el), MATLAB Function10/1(sin_theta_el), MATLAB Function1/1(sin_theta_el), MATLAB Function/1(sin_theta_el)
  cos_theta_el1/1 -> MATLAB Function9/2(cos_theta_el), MATLAB Function8/2(cos_theta_el), MATLAB Function7/2(cos_theta_el), MATLAB Function6/2(cos_theta_el), MATLAB Function5/2(cos_theta_el), MATLAB Function4/2(cos_theta_el), MATLAB Function3/2(cos_theta_el), MATLAB Function2/2(cos_theta_el), MATLAB Function15/2(cos_theta_el), MATLAB Function14/2(cos_theta_el), MATLAB Function13/2(cos_theta_el), MATLAB Function12/2(cos_theta_el), MATLAB Function11/2(cos_theta_el), MATLAB Function10/2(cos_theta_el), MATLAB Function1/2(cos_theta_el), MATLAB Function/2(cos_theta_el)

== system gm_test_phase_voltages_without_delays/Phase_voltages_per_switching_state1/Detect Rise Positive/Positive ==
  u : Inport  OutDataTypeStr=boolean  SampleTime=1e-08
  Compare : RelationalOperator  Operator=>  OutDataTypeStr=boolean  ZeroCross=off
  Constant : Constant  DisableCoverage=on  Value=0  OutDataTypeStr=Inherit: Inherit via back propagation  SampleTime=-1  PreserveConstantTs=on
  y : Outport  SampleTime=1e-08
  wires:
  Compare/1 -> y/1
  Constant/1 -> Compare/2
  u/1 -> Compare/1
